simulink model "Simplified7DOF"  (R2019b)
settings: Solver=VariableStepAuto  StartTime=0.0  StopTime=10.0  RelTol=1e-3
settings Model: Creator=yeyuan  LastModifiedBy=yeyuan

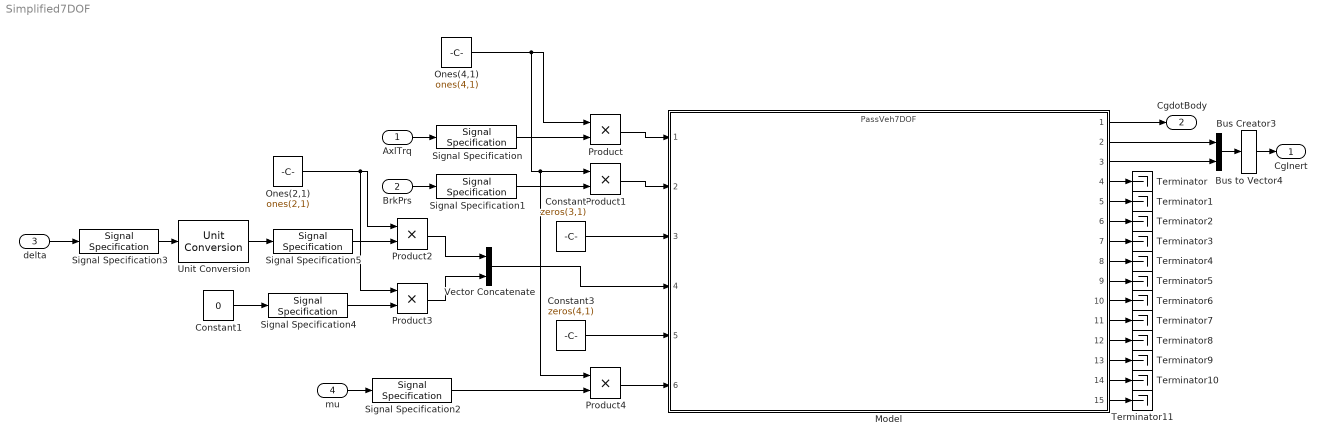
== system Simplified7DOF ==
  AxlTrq : Inport
  BrkPrs : Inport  Port=2
  delta : Inport  Port=3
  mu : Inport  Port=4
  Bus Creator3 : BusCreator  Inputs=2
  Bus to Vector4 : BusToVector
  Constant : Constant  Value=zeros(3,1)
  Constant1 : Constant  Value=0
  Constant3 : Constant  Value=zeros(4,1)
  Model : ModelReference  ModelNameDialog=PassVeh7DOF.slx  SimulationMode=Normal  ModelReferenceVersion=1.144
  Ones(2,1) : Constant  Value=ones(2,1)  OutDataTypeStr=Inherit: Inherit via back propagation
  Ones(4,1) : Constant  Value=ones(4,1)  OutDataTypeStr=Inherit: Inherit via back propagation
  Product{,1..4} (5 alike) : Product
  Signal Specification : SignalSpecification  Unit=N*m
  Signal Specification1 : SignalSpecification  Unit=Pa
  Signal Specification2 : SignalSpecification  Unit=1
  Signal Specification3 : SignalSpecification  Unit=deg
  Signal Specification4 : SignalSpecification  Unit=rad
  Signal Specification5 : SignalSpecification  Unit=rad
  Terminator{,1..11} (12 alike) : Terminator
  Unit Conversion : UnitConversion
  Vector Concatenate : Concatenate
  CgInert : Outport
  CgdotBody : Outport  Port=2
  wires:
  Constant3/1 -> Model/5
  Constant/1 -> Model/3
  mu/1 -> Signal Specification2/1
  AxlTrq/1 -> Signal Specification/1
  BrkPrs/1 -> Signal Specification1/1
  Model/2 -> Bus Creator3/1
  Model/3 -> Bus Creator3/2
  Model/1 -> CgdotBody/1
  delta/1 -> Signal Specification3/1
  Signal Specification3/1 -> Unit Conversion/1
  Constant1/1 -> Signal Specification4/1
  Unit Conversion/1 -> Signal Specification5/1
  Bus Creator3/1 -> Bus to Vector4/1
  Bus to Vector4/1 -> CgInert/1
  Model/4 -> Terminator/1
  Model/5 -> Terminator1/1
  Model/6 -> Terminator2/1
  Model/7 -> Terminator3/1
  Model/8 -> Terminator4/1
  Model/9 -> Terminator5/1
  Model/10 -> Terminator6/1
  Model/11 -> Terminator7/1
  Model/12 -> Terminator8/1
  Model/13 -> Terminator9/1
  Model/14 -> Terminator10/1
  Model/15 -> Terminator11/1
  Ones(4,1)/1 -> Product4/1, Product1/1, Product/1
  Signal Specification/1 -> Product/2
  Product/1 -> Model/1
  Signal Specification1/1 -> Product1/2
  Product1/1 -> Model/2
  Signal Specification5/1 -> Product2/2
  Ones(2,1)/1 -> Product3/1, Product2/1
  Signal Specification4/1 -> Product3/2
  Product2/1 -> Vector Concatenate/1
  Product3/1 -> Vector Concatenate/2
  Vector Concatenate/1 -> Model/4
  Product4/1 -> Model/6
  Signal Specification2/1 -> Product4/2
